simulink model "FIR_filter"  (R2020a)
settings: Solver=VariableStepAuto  StartTime=0.0  StopTime=20  RelTol=1e-3
libraries: dspsrcs4 x1
settings Model: Creator=Admin  LastModifiedBy=Admin

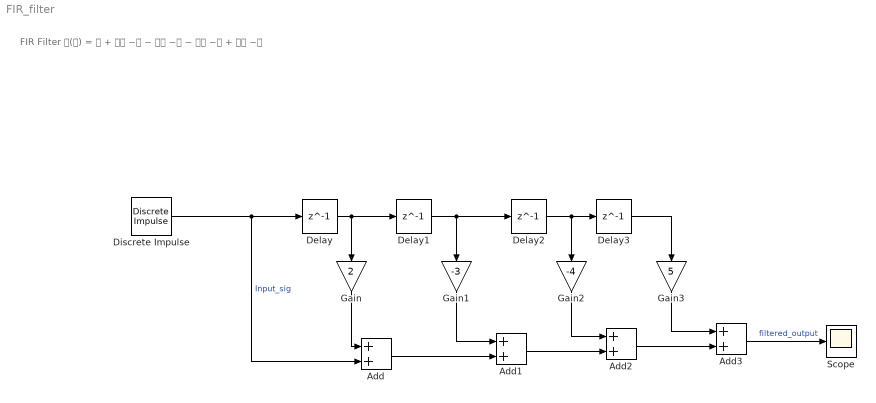
== system FIR_filter ==
  note: FIR Filter
      |
      | 𝐇(𝐳) = 𝟏 + 𝟐𝐳 −𝟏 − 𝟑𝐳 −𝟐 − 𝟒𝐳 −𝟑 + 𝟓𝐳 −𝟒
  Add{,1..3} (4 alike) : Sum
  Delay{,1..3} (4 alike) : Delay  DelayLength=1
  Discrete Impulse : dspsrcs4/Discrete  Impulse  Delay=0  SampleTime=1  FrameSample=1  OutputFrames=off  dataType=double  isSigned=on  wordLen=16  udDataType=sfix(16)  fracBitsMode=Best precision  numFracBits=15  OutDataTypeStr=double  LastOutDataTypeStr=double
  Gain : Gain  Gain=2
  Gain1 : Gain  Gain=-3
  Gain2 : Gain  Gain=-4
  Gain3 : Gain  Gain=5
  Scope : Scope
  wires:
  Discrete Impulse/1 -> Add/2, Delay/1  "Input_sig"
  Delay/1 -> Gain/1, Delay1/1
  Delay1/1 -> Gain1/1, Delay2/1
  Delay2/1 -> Gain2/1, Delay3/1
  Delay3/1 -> Gain3/1
  Gain/1 -> Add/1
  Gain1/1 -> Add1/1
  Add/1 -> Add1/2
  Add1/1 -> Add2/2
  Gain2/1 -> Add2/1
  Add2/1 -> Add3/2
  Gain3/1 -> Add3/1
  Add3/1 -> Scope/1  "filtered_output"
